simulink model "testEmplanner_cs_old"  (R2021b)
settings: Solver=ode5  StartTime=0.0  StopTime=60  FixedStep=1/1000  RelTol=1e-3
PreLoadFcn:
  | mbxruntime.callbacks.PreLoadFcn(bdroot);
PostLoadFcn:
  | mbxruntime.callbacks.PostLoadFcn(bdroot);
InitFcn:
  | mbxruntime.callbacks.InitFcn(bdroot);
StartFcn:
  | mbxruntime.callbacks.StartFcn(bdroot);
StopFcn:
  | mbxruntime.callbacks.StopFcn(bdroot);
model workspace (MAT data in the model file):
  mbox_table : object (value not decoded)
  model_closed = 0
  sim_status = 0
values from neighbouring files (symbols this model uses):
  c_factor = 43.75    [emplanner_init.m]
  cf = -175016    [emplanner_init.m]
  cr = -130634    [emplanner_init.m]
  global_path_x = [-1.1448 -0.145417744933 0.852705365581 1.84955224935 2.84511712279 3.83939835808 4.83239585569 5.82411007764 6.81454169183 7.80369144113 8.79156009523 9.77814843293 ... (3001 elements, 3001x1)]    [global_path.mat]
  global_path_y = [14.6488 14.6488 14.6488 14.6488 14.6488 14.6488 14.6488 14.6488 14.6488 14.6488 14.6488 14.6488 ... (3001 elements, 3001x1)]    [global_path.mat]
  KD_PID_distance = 0.0    (= 0)    [emplanner_init.m]
  KD_PID_speed = 0    [emplanner_init.m]
  KI_PID_distance = 0.0    (= 0)    [emplanner_init.m]
  KI_PID_speed = 0    [emplanner_init.m]
  KP_PID_distance = 0.5    [emplanner_init.m]
  KP_PID_speed = 1.8    [emplanner_init.m]
  la = 1.265    [emplanner_init.m]
  lb = 2.947-1.265    (= 1.682)    [emplanner_init.m]
  LQR_K1 = k(:,1)'    [emplanner_init.m]
  LQR_K2 = k(:,2)'    [emplanner_init.m]
  LQR_K3 = k(:,3)'    [emplanner_init.m]
  LQR_K4 = k(:,4)'    [emplanner_init.m]
  m = 2020    [emplanner_init.m]
  rack_displacement = [-39.14 , -37.2 , -35.29 , -33.43 , -31.6 , -29.81 , -28.06 , -26.34 , -24.66 ,      -23.01 , -21.38 , -19.79 , -18.23 , -16.69 , -15.18 , -13.7 , -12.23 , -10.8 , -9.38 , -7.98 ,     -6.61 , -5.25 , -3.91 , -2.59 , -1.29 , 0 , 1.27 , 2.54 , 3.78 , 5.02 , 6.24 , 7.46 , 8.66 ,      9.86 , 11.05 , 12.24 , 13.41 , 14.59 , 15.76 , 16.92 , 18.09 , 19.25 , 20.42 , 21.59 , 22.76 ,      23.93 , 25.11 , 26 ...(+26 chars)    [emplanner_init.m]
  right_wheel_ground = [-70 ,-67.2 , -64.4 , -61.6 , -58.8 , -56 , -53.2 , -50.4 , -47.6 , -44.8 , -42 ,      -39.2 , -36.4 , -33.6 , -30.8 , -28 , -25.2 , -22.4 , -19.6 , -16.8 , -14 , -11.2 , -8.4 , -5.6 ,      -2.8 , 0 , 2.8 , 5.6 , 8.4 , 11.2 , 14 , 16.8 , 19.6 , 22.4 , 25.2 , 28 , 30.8 , 33.6 , 36.4 ,      39.2 , 42 , 44.8 , 47.6 , 50.4 , 53.2 , 56 , 58.8 , 61.6 , 64.4 , 67.2 , 70 ]    [emplanner_init.m]
  vx_break_point = zeros(1,5000)    [emplanner_init.m]
undefined symbols (not defined in the file or in its folder): aubr, DiscIntNeverNeededParam, tablebr, vubr, warningInitialVelocity, x0
libraries: simulink x19, PreScanSimulinkLibrary x17, simulink_extras x6, Solver_SF x1
(part 11 of 14)

== matlab function testEmplanner_cs_old/Audi_A8_Sedan_1/decision&planning module/EM Planner/obs/MATLAB Function ==
  data: obs_x_set_gcs input; static_obs_x_set output; obs_y_set_gcs input; obs_heading_set_gcs input; obs_velocity_set_gcs input; static_obs_y_set output; dynamic_obs_x_set output; dynamic_obs_y_set output; dynamic_obs_vx_set output; dynamic_obs_vy_set output
function [static_obs_x_set,static_obs_y_set,dynamic_obs_x_set,dynamic_obs_y_set,dynamic_obs_vx_set,dynamic_obs_vy_set]...
	= fcn(obs_x_set_gcs,obs_y_set_gcs,obs_heading_set_gcs,obs_velocity_set_gcs)
%该函数将分类静态障碍物和动态障碍物
%输出初始化
n = 32;
static_obs_x_set = ones(n,1) * nan; 
static_obs_y_set = ones(n,1) * nan; 
dynamic_obs_x_set = ones(n,1) * nan; 
dynamic_obs_y_set = ones(n,1) * nan; 
dynamic_obs_vx_set = ones(n,1) * nan; 
dynamic_obs_vy_set = ones(n,1) * nan; 

count_static = 1;
count_dynamic = 1;

for i = 1 : length(obs_x_set_gcs)
	if isnan(obs_velocity_set_gcs(i))
		break;
	end
	if abs(obs_velocity_set_gcs(i)) < 0.1 
		static_obs_x_set(count_static) = obs_x_set_gcs(i); 
		static_obs_y_set(count_static) = obs_y_set_gcs(i);
		count_static = count_static + 1;
	else
		dynamic_obs_x_set(count_dynamic) = obs_x_set_gcs(i); 
		dynamic_obs_y_set(count_dynamic) = obs_y_set_gcs(i);
		dynamic_obs_vx_set(count_dynamic) = obs_velocity_set_gcs(i)*cos(obs_heading_set_gcs(i));
		dynamic_obs_vy_set(count_dynamic) = obs_velocity_set_gcs(i)*sin(obs_heading_set_gcs(i));
		count_dynamic = count_dynamic + 1;
	end
end

== matlab function testEmplanner_cs_old/Audi_A8_Sedan_1/decision&planning module/EM Planner/obs/MATLAB Function5 ==
  data: x_set input; match_point_index_set output; y_set input; frenet_path_x input; frenet_path_y input; frenet_path_heading input; frenet_path_kappa input; proj_x_set output; proj_y_set output; proj_heading_set output; proj_kappa_set output
function [match_point_index_set,proj_x_set,proj_y_set,proj_heading_set,proj_kappa_set] = ...
	fcn(x_set,y_set,frenet_path_x,frenet_path_y,frenet_path_heading,frenet_path_kappa)
	
%该函数将批量计算x_set,y_set中(x,y) 在frenet坐标系下的投影信息
%输入： x_set，y_set 待投影的点的集合
	%x_set,y_set,frenet_path_x,frenet_path_y,frenet_path_heading,frenet_path_kappa
	%曲线在直角坐标系下的x,y,heading,kappa
%输出：math_point_index_set 匹配点在frenet_path下的编号的集合（即从全局路径的第一个点开始数，第几个点是匹配点）

%由于事先不知道x_set中有多少个点需要投影，因此事先声明一个最大数量的点作为缓冲

n = 128;
%并且不知道投影点的数量，所以也不知道输出的数量，因此输出也要做缓冲，用nan表示不存在的点
%初始化输出最多为128个点。
%输出初始化
match_point_index_set = ones(n,1) * nan;
proj_x_set = ones(n,1) * nan;
proj_y_set = ones(n,1) * nan;
proj_heading_set = ones(n,1) * nan;
proj_kappa_set = ones(n,1) * nan;

%找匹配点，需要利用上一个周期的结果作为下一个周期遍历的起点，因此需要声明两个全局变量
persistent is_first_run;
persistent pre_match_point_index_set;
persistent pre_frenet_path_x;
persistent pre_frenet_path_y;
persistent pre_frenet_path_heading;
persistent pre_frenet_path_kappa;

%算法主函数入口

if isempty(is_first_run)
	% 该if分支表示函数首次运行
	is_first_run = 0; %赋值
	pre_frenet_path_x = frenet_path_x;
	pre_frenet_path_y = frenet_path_y;
	pre_frenet_path_heading = frenet_path_heading;
	pre_frenet_path_kappa = frenet_path_kappa;
	%记录首次运行计算的匹配点的结果供下个周期运行，先初始化
	pre_match_point_index_set = ones(n,1) * nan;
	
	%对x_set,y_set的点做遍历，找到他们的匹配点
	for i = 1 : length(x_set)
        if isnan(x_set(i))
            break;
        end
		%首次运行时，没有任何提示，只能从frenet_path的第一个点开始找
		start_search_index = 1;
		%声明increa_count,用于表示在遍历时distance连续增大的次数
		increase_count = 0;
		%开始遍历
		min_distance = inf;
		for j = start_search_index : length(frenet_path_x)
			distance = (x_set(i) - frenet_path_x(j))^2 + (y_set(i) - frenet_path_y(j))^2;
			%处理最小值
			if distance < min_distance
				min_distance = distance;
				match_point_index_set(i) = j; %math_point_index_set存放匹配点的序号
				increase_count = 0;
			else
				increase_count = increase_count + 1;
			end
			% 如果连续distanc增加50次,就不要再遍历了，节省时间
			if increase_count > 50 
				break;
			end	
		end
		%如何通过匹配点计算投影点，参考《自动驾驾驶控制算法第七讲》
		%或者《自动驾驶决策规划算法》第一章第三节
		
		%取出匹配点的编号
		match_point_index = match_point_index_set(i);
		
		%取出匹配点信息
		match_point_x = frenet_path_x(match_point_index);
		match_point_y = frenet_path_y(match_point_index);
		match_point_heading = frenet_path_heading(match_point_index);
		match_point_kappa = frenet_path_kappa(match_point_index);
		
		% 计算匹配点的位置向量和方向向量
		vector_match_point = [match_point_x;match_point_y];%位置向量
		vector_match_point_direction = [cos(match_point_heading);sin(match_point_heading)];%方向向量，全局坐标系下（大地坐标系）
		
		%声明待投影点的位矢
		vector_r = [x_set(i);y_set(i)];
		
		%通过匹配点计算投影点
		vector_d = vector_r - vector_match_point;
		ds = vector_d' * vector_match_point_direction;
		vector_proj_point = vector_match_point + vector_match_point_direction *ds;
		proj_heading = match_point_heading + match_point_kappa * ds;
		proj_kappa = match_point_kappa;
		
		%计算结果输出 
		proj_x_set(i) = vector_proj_point(1);
		proj_y_set(i) = vector_proj_point(2);
		proj_heading_set(i) = proj_heading;
		proj_kappa_set(i) = proj_kappa;
	end
	
	%匹配点的计算结果保存，供下一个周期使用
	pre_match_point_index_set = match_point_index_set;
else
	% 此分支不是首次运行
	
	%对每个x_set上的点做处理
	for i = 1 : length(x_set)
		%不是首次运行，对于点x_set(i),y_set(i)来说，start_search_index = pre_match_point_index_set(i)
		start_search_index = pre_match_point_index_set(i);%上个周期匹配点的编号作为本周期搜索的起点
		
        %
        % 对于障碍物的检测而言，当感知第一次检测到障碍物时，算法并不是首次运行，此时
        % pre_match_point_set的值是nan，如果还用上一个时刻的结果作为本周期搜索的起点
        % 必然会出问题，所以要修改
        % 声明 increase_count_limit
        increase_count_limit = 5;
        if isnan(start_search_index)
	        % 没有上个周期的结果，那么就不能只检查5次
	        increase_count_limit = 50;
	        % 搜索的起点也要设为 1
	        start_search_index = 1;
        end
		%声明increa_count,用于表示在遍历时distance连续增大的次数
		increase_count = 0;
		%开始遍历
		
		%这里多了一个步骤，判断遍历的方向
		%计算上个周期匹配点的位失
		vector_pre_match_point = [pre_frenet_path_x(start_search_index); pre_frenet_path_y(start_search_index)];
		vector_pre_match_point_direction = ...
			[cos(pre_frenet_path_heading(start_search_index));sin(pre_frenet_path_heading(start_search_index))];
		
		% 判断遍历的方向
		flag = ([x_set(i);y_set(i)] - vector_pre_match_point)' * vector_pre_match_point_direction;
		
		min_distance = inf;
		
		if flag > 0.001 
			for j = start_search_index : length(frenet_path_x)
				distance = (x_set(i) - frenet_path_x(j))^2 + (y_set(i) - frenet_path_y(j))^2;
				%处理最小值
				if distance < min_distance
					min_distance = distance;
					match_point_index_set(i) = j; %math_point_index_set存放匹配点的序号
					increase_count = 0;
				else
					increase_count = increase_count + 1;
				end
				% 如果连续distanc增加increase_count_limit次,就不要再遍历了，节省时间
				if increase_count > increase_count_limit
					break;
				end
			end
		elseif flag < -0.001
			for j = start_search_index :-1: 1
				distance = (x_set(i) - frenet_path_x(j))^2 + (y_set(i) - frenet_path_y(j))^2;
				%处理最小值
				if distance < min_distance
					min_distance = distance;
					match_point_index_set(i) = j; %math_point_index_set存放匹配点的序号
					increase_count = 0;
				else
					increase_count = increase_count + 1;
				end
				% 如果连续distanc增加50次,就不要再遍历了，节省时间
				if increase_count > increase_count_limit 
					break;
				end
			end
		else
			match_point_index_set(i) = start_search_index;
		end
			
		%如何通过匹配点计算投影点，参考《自动驾驾驶控制算法第七讲》
		%或者《自动驾驶决策规划算法》第一章第三节
		
		%取出匹配点的编号
		match_point_index = match_point_index_set(i);
		
		%取出匹配点信息
		match_point_x = frenet_path_x(match_point_index);
		match_point_y = frenet_path_y(match_point_index);
		match_point_heading = frenet_path_heading(match_point_index);
		match_point_kappa = frenet_path_kappa(match_point_index);
		
		% 计算匹配点的位置向量和方向向量
		vector_match_point = [match_point_x;match_point_y];%位置向量
		vector_match_point_direction = [cos(match_point_heading);sin(match_point_heading)];%方向向量
		
		%声明待投影点的位矢
		vector_r = [x_set(i);y_set(i)];
		
		%通过匹配点计算投影点
		vector_d = vector_r - vector_match_point;
		ds = vector_d' * vector_match_point_direction;
		vector_proj_point = vector_match_point + ds * vector_match_point_direction;
		proj_heading = match_point_heading + match_point_kappa * ds;
		proj_kappa = match_point_kappa;
		
		%计算结果输出 
		proj_x_set(i) = vector_proj_point(1);
		proj_y_set(i) = vector_proj_point(2);
		proj_heading_set(i) = proj_heading;
		proj_kappa_set(i) = proj_kappa;
	end
	
	%匹配点的计算结果保存，供下一个周期使用
	pre_match_point_index_set = match_point_index_set;
	pre_frenet_path_x = frenet_path_x;
	pre_frenet_path_y = frenet_path_y;
	pre_frenet_path_heading = frenet_path_heading;
	pre_frenet_path_kappa = frenet_path_kappa;
end

== matlab function testEmplanner_cs_old/Audi_A8_Sedan_1/decision&planning module/EM Planner/obs/obs filter ==
  data: host_x input; obs_x_set_final output; host_y input; host_heading_xy input; obs_x_set_gcs input; obs_y_set_gcs input; obs_heading_set_gcs input; obs_velocity_set_gcs input; obs_y_set_final output; obs_velocity_set_final output; obs_heading_set_final output
function [obs_x_set_final,obs_y_set_final,obs_velocity_set_final,obs_heading_set_final] = fcn(host_x,host_y,host_heading_xy, ...
	obs_x_set_gcs,obs_y_set_gcs,obs_heading_set_gcs,obs_velocity_set_gcs)
% 该函数将筛选障碍物，纵向[-10,60] 横向[-25,25]的障碍物才会被考虑
% 该函数只是一种单车道的临时办法，考虑到多车道情况，即使障碍物距离较远也应该考虑
% EM Planner 完全体是多车道并行计算的，每个车道都生成参考线后并行计算出多条轨迹，然后再选择最优轨迹作为输出
% 传感器最多可以识别32个障碍物
n = 32;
% 输出初始化

obs_x_set_final = ones(n,1)*nan;
obs_y_set_final = ones(n,1)*nan;
obs_velocity_set_final = ones(n,1)*nan;
obs_heading_set_final = ones(n,1)*nan;
count = 1;
for i = 1 : length(obs_x_set_gcs)
	if isnan(obs_x_set_gcs(i))
		break;
	end
	%自车的heading的方向向量与法向量
	tor = [cos(host_heading_xy);sin(host_heading_xy)];
	nor = [-sin(host_heading_xy);cos(host_heading_xy)];
	% 障碍物与自车的距离向量
	vetor_obs = [obs_x_set_gcs(i);obs_y_set_gcs(i)] - [host_x;host_y];
	% 障碍物距离自车的纵向距离
	lon_distance = vetor_obs' * tor;
	% 障碍物距离自车的横向距离
	lat_distance = vetor_obs' * nor;
	
	if (lon_distance < 60) && (lon_distance > -10) && (lat_distance > -25) && (lat_distance < 25)
		obs_x_set_final(count) = obs_x_set_gcs(i);
		obs_y_set_final(count) = obs_y_set_gcs(i);
		obs_heading_set_final(count) = obs_heading_set_gcs(i);
		obs_velocity_set_final(count) = obs_velocity_set_gcs(i);
		count = count + 1;
	end
end

== matlab function testEmplanner_cs_old/Audi_A8_Sedan_1/decision&planning module/EM Planner/path and speed merge ==
  data: s input; trajectory_x output; s_dot input; s_dot2 input; relative_time input; current_time input; path_s input; trajectory_x_init input; trajectory_y_init input; trajectory_heading_init input; trajectory_kappa_init input; trajectory_y output; trajectory_heading output; trajectory_kappa output; trajectory_speed output; trajectory_accel output; trajectory_time output
function [trajectory_x,trajectory_y,trajectory_heading,trajectory_kappa,trajectory_speed,trajectory_accel,trajectory_time] = ...
    fcn(s,s_dot,s_dot2,relative_time,current_time,path_s,trajectory_x_init,trajectory_y_init,trajectory_heading_init,trajectory_kappa_init)
% 该函数将合并path和speed
% 由于path 是 60个点，speed 有 401个点，合并后，path和speed有401个点，因此需要做插值
n = 401;
trajectory_x = zeros(n,1);
trajectory_y = zeros(n,1);
trajectory_heading = zeros(n,1);
trajectory_kappa = zeros(n,1);
trajectory_speed = zeros(n,1);

trajectory_accel = zeros(n,1);
index = 1;
% 由于trajectory_x_init中不是所有的值都有效，(有nan) 所以要找到有效值的范围
while ~isnan(trajectory_x_init(index)) 
    index = index + 1;
end
index = index - 1;
trajectory_time = zeros(n,1);
for i = 1:n-1
    %interp1 线性插值
    % 若 x = [1,2] y = [3,4]
    %interp1(x,y,1.5) 会得到3.5
    %interp1 的缺点是 在端点或超过端点的，结果为nan
    % interp1(x,y,2) 不会等于4 而是会等于nan
    % interp1(x,y,6) 也会等于nan，所以在端点处要单独处理
    trajectory_x(i) = interp1(path_s(1:index),trajectory_x_init(1:index),s(i));
    trajectory_y(i) = interp1(path_s(1:index),trajectory_y_init(1:index),s(i));
    trajectory_heading(i) = interp1(path_s(1:index),trajectory_heading_init(1:index),s(i));
    trajectory_kappa(i) = interp1(path_s(1:index),trajectory_kappa_init(1:index),s(i));
    trajectory_time(i) = relative_time(i) + current_time;%速度规划会得到相对时间，转换成绝对时间
    trajectory_speed(i) = s_dot(i);
    trajectory_accel(i) = s_dot2(i);
end
% 端点单独处理
trajectory_x(end) = trajectory_x_init(end);
trajectory_y(end) = trajectory_y_init(end);
trajectory_heading(end) = trajectory_heading_init(end);
trajectory_kappa(end) = trajectory_kappa_init(end);
trajectory_time(end) = relative_time(end) + current_time;
trajectory_speed(end) = s_dot(end);
trajectory_accel(end) = s_dot2(end);

== matlab function testEmplanner_cs_old/Audi_A8_Sedan_2/PathFollower_Preview_1/LateralController/Calculate delta steering error/eml_delta_steering_error ==
  data: v_x_vehicle input; v_x_vehicle_Min input; t_Preview_LatCtrl input; delta_steeringwheeltotal output; v_y_vehicle input; yawrate_vehicle input; CorneringStiffness_Tyres_Front input; CorneringStiffness_Tyres_Rear input; m_vehicle_total input; inertia_z_vehicle_total input; e_Lat input size=10; Pos_x_CoG_Vehicle input; wheelbase input; RefreshCounter parameter
function delta_steeringwheeltotal = eml_delta_steering_error(v_x_vehicle,v_x_vehicle_Min,t_Preview_LatCtrl,v_y_vehicle,yawrate_vehicle,CorneringStiffness_Tyres_Front,CorneringStiffness_Tyres_Rear,m_vehicle_total,inertia_z_vehicle_total,e_Lat,Pos_x_CoG_Vehicle,wheelbase,RefreshCounter)

delta_steeringwheeltotal = emlfcn_delta_steering_error(v_x_vehicle,v_x_vehicle_Min,t_Preview_LatCtrl,v_y_vehicle,yawrate_vehicle,CorneringStiffness_Tyres_Front,CorneringStiffness_Tyres_Rear,m_vehicle_total,inertia_z_vehicle_total,e_Lat,Pos_x_CoG_Vehicle,wheelbase,RefreshCounter);

% end function

== matlab function testEmplanner_cs_old/Audi_A8_Sedan_1/decision&planning module/EM Planner/plot ==
  data: dp_s input; dp_l input; qp_s input; qp_l input; l_min input; l_max input; obs_s_set input; obs_l_set input; start_s input; start_l input; start_dl input
function  fcn(dp_s,dp_l,qp_s,qp_l,l_min,l_max,obs_s_set,obs_l_set,start_s,start_l,start_dl)
coder.extrinsic("plot","axis","figure","drawnow","cla","fill");

obs_length = 5;
obs_width = 2;
host_l = 6;
host_w = 1.63;
cla;
host_p1_l = start_l + sin(atan(start_dl)) * host_l /2 + host_w/2 * cos(atan(start_dl));
host_p1_s = start_s + cos(atan(start_dl)) * host_l /2 - host_w/2 * sin(atan(start_dl));
host_p2_l = start_l + sin(atan(start_dl)) * host_l /2 - host_w/2 * cos(atan(start_dl));
host_p2_s = start_s + cos(atan(start_dl)) * host_l /2 + host_w/2 * sin(atan(start_dl));
host_p3_l = start_l - sin(atan(start_dl)) * host_l /2 + host_w/2 * cos(atan(start_dl));
host_p3_s = start_s - cos(atan(start_dl)) * host_l /2 - host_w/2 * sin(atan(start_dl));
host_p4_l = start_l - sin(atan(start_dl)) * host_l /2 - host_w/2 * cos(atan(start_dl));
host_p4_s = start_s - cos(atan(start_dl)) * host_l /2 + host_w/2 * sin(atan(start_dl));
host_area_x = [host_p1_s;host_p2_s;host_p4_s;host_p3_s];
host_area_y = [host_p1_l;host_p2_l;host_p4_l;host_p3_l];
fill(host_area_x,host_area_y,[0 1 1]);
hold on
plot(dp_s,dp_l,'r');

plot(qp_s,qp_l,'b');
plot(dp_s,l_min,dp_s,l_max);
axis([-8 70 -10 10]);

for i = 1:length(obs_s_set)
    if isnan(obs_s_set(i))
        break;
    end
    obs_p1_s = obs_s_set(i) + obs_length/2;
    obs_p1_l = obs_l_set(i) + obs_width/2;
    obs_p2_s = obs_s_set(i) + obs_length/2;
    obs_p2_l = obs_l_set(i) - obs_width/2;
    obs_p3_s = obs_s_set(i) - obs_length/2;
    obs_p3_l = obs_l_set(i) + obs_width/2;
    obs_p4_s = obs_s_set(i) - obs_length/2;
    obs_p4_l = obs_l_set(i) - obs_width/2;
    obs_area_s = [obs_p1_s;obs_p2_s;obs_p4_s;obs_p3_s];
    obs_area_l = [obs_p1_l;obs_p2_l;obs_p4_l;obs_p3_l];
    fill(obs_area_s,obs_area_l,[0 0 0]);
end

== matlab function testEmplanner_cs_old/Audi_A8_Sedan_1/decision&planning module/EM Planner/simple speed qp planning ==
  data: plan_start_s_dot input; s_init output; plan_start_s_dot2 input; s_end input; recommend_T input; s_dot_init output; s_dot2_init output; relative_time_init output
function [s_init,s_dot_init,s_dot2_init,relative_time_init] = fcn(plan_start_s_dot,plan_start_s_dot2,s_end,recommend_T)
%简单速度二次规划
coder.extrinsic("quadprog")
n = 51;
s_init = zeros(n,1);
s_dot_init = zeros(n,1);
s_dot2_init = zeros(n,1);
relative_time_init = zeros(n,1);

Aeq = zeros(3*n,2*n - 2);
beq = zeros(2*n - 2,1);
lb = ones(3*n,1);
ub = lb;
dt = recommend_T/(n-1);
A_sub =[1,0;
        dt,1;
        (1/3)*dt^2,(1/2)*dt;
        -1,0;
        0,-1;
        (1/6)*dt^2,dt/2];
for i = 1:n - 1
    Aeq(3*i-2:3*i+3,2*i-1:2*i) = A_sub;
end

for i = 1:n
   lb(3*i - 2) = -inf;
   lb(3*i - 1) = 0;
   lb(3*i) = -8;
   ub(3*i - 2) = inf;
   ub(3*i - 1) = 50;
   ub(3*i) = 2;
end
lb(1) = 0;
lb(2) = plan_start_s_dot;
lb(3) = plan_start_s_dot2;
ub(1) = lb(1);
ub(2) = lb(2);
ub(3) = lb(3);
lb(3*n - 2) = s_end;
ub(3*n - 2) = s_end;
A3 = zeros(3*n,3*n);
A4 = zeros(3*n,n - 1);
A4_sub =[0;0;1;0;0;-1];
for i = 1:n - 1
   A3(3*i,3*i) = 1;
   A4(3*i-2:3*i+3,i:i) = A4_sub;
end
A3(3*n,3*n) = 1;
H = A3 + 100*(A4*A4');
H = 2*H;
f = zeros(3*n,1);
X = quadprog(H,f,[],[],Aeq',beq,lb,ub);
for i = 1:n
   s_init(i) = X(3*i - 2);
   s_dot_init(i) = X(3*i - 1);
   s_dot2_init(i) = X(3*i);
   relative_time_init(i) = (i - 1)*dt;
end

== matlab function testEmplanner_cs_old/Audi_A8_Sedan_1/decision&planning module/EM Planner/stitch trajectory ==
  data: trajectory_x input; trajectory_x_final output; trajectory_y input; trajectory_heading input; trajectory_kappa input; trajectory_speed input; trajectory_accel input; trajectory_time input; stitch_x input; stitch_y input; stitch_heading input; stitch_kappa input; stitch_speed input; stitch_accel input; stitch_time input; trajectory_y_final output; trajectory_heading_final output; trajectory_kappa_final output; trajectory_speed_final output; trajectory_accel_final output; trajectory_time_final output
function [trajectory_x_final,trajectory_y_final,trajectory_heading_final,trajectory_kappa_final,...
          trajectory_speed_final,trajectory_accel_final,trajectory_time_final] = fcn(trajectory_x,...
          trajectory_y,trajectory_heading,trajectory_kappa,trajectory_speed,trajectory_accel,trajectory_time,...
          stitch_x,stitch_y,stitch_heading,stitch_kappa,stitch_speed,stitch_accel,stitch_time)
% 轨迹拼接，把stitch trajectory 拼到规划完成的轨迹上
n = 401 + 20;
trajectory_x_final = zeros(n,1);
trajectory_y_final = zeros(n,1);
trajectory_heading_final = zeros(n,1);
trajectory_kappa_final = zeros(n,1);
trajectory_speed_final = zeros(n,1);
trajectory_accel_final = zeros(n,1);
trajectory_time_final = zeros(n,1);

trajectory_x_final = [stitch_x;trajectory_x];
trajectory_y_final = [stitch_y;trajectory_y];
trajectory_heading_final = [stitch_heading;trajectory_heading];
trajectory_kappa_final = [stitch_kappa;trajectory_kappa];
trajectory_speed_final = [stitch_speed;trajectory_speed];
trajectory_accel_final = [stitch_accel;trajectory_accel];
trajectory_time_final = [stitch_time;trajectory_time];

== matlab function testEmplanner_cs_old/Audi_A8_Sedan_1/decision&planning module/EM Planner2/simple speed qp planning ==
  data: plan_start_s_dot input; s_init output; plan_start_s_dot2 input; s_end input; recommend_T input; s_dot_init output; s_dot2_init output; relative_time_init output
function [s_init,s_dot_init,s_dot2_init,relative_time_init] = fcn(plan_start_s_dot,plan_start_s_dot2,s_end,recommend_T)
%简单速度二次规划
coder.extrinsic("quadprog")
n = 51;
s_init = zeros(n,1);
s_dot_init = zeros(n,1);
s_dot2_init = zeros(n,1);
relative_time_init = zeros(n,1);

Aeq = zeros(3*n,2*n - 2);
beq = zeros(2*n - 2,1);
lb = ones(3*n,1);
ub = lb;
dt = recommend_T/(n-1);
A_sub =[1,0;
        dt,1;
        (1/3)*dt^2,(1/2)*dt;
        -1,0;
        0,-1;
        (1/6)*dt^2,dt/2];
for i = 1:n - 1
    Aeq(3*i-2:3*i+3,2*i-1:2*i) = A_sub;
end

for i = 1:n
   lb(3*i - 2) = -inf;
   lb(3*i - 1) = 0;
   lb(3*i) = -8;
   ub(3*i - 2) = inf;
   ub(3*i - 1) = 50;
   ub(3*i) = 2;
end
lb(1) = 0;
lb(2) = plan_start_s_dot;
lb(3) = plan_start_s_dot2;
ub(1) = lb(1);
ub(2) = lb(2);
ub(3) = lb(3);
lb(3*n - 2) = s_end;
ub(3*n - 2) = s_end;
A3 = zeros(3*n,3*n);
A4 = zeros(3*n,n - 1);
A4_sub =[0;0;1;0;0;-1];
for i = 1:n - 1
   A3(3*i,3*i) = 1;
   A4(3*i-2:3*i+3,i:i) = A4_sub;
end
A3(3*n,3*n) = 1;
H = A3 + 100*(A4*A4');
H = 2*H;
f = zeros(3*n,1);
X = quadprog(H,f,[],[],Aeq',beq,lb,ub);
for i = 1:n
   s_init(i) = X(3*i - 2);
   s_dot_init(i) = X(3*i - 1);
   s_dot2_init(i) = X(3*i);
   relative_time_init(i) = (i - 1)*dt;
end

== matlab function testEmplanner_cs_old/Audi_A8_Sedan_1/decision&planning module/EM Planner2/stitch trajectory ==
  data: trajectory_x input; trajectory_x_final output; trajectory_y input; trajectory_heading input; trajectory_kappa input; trajectory_speed input; trajectory_accel input; trajectory_time input; stitch_x input; stitch_y input; stitch_heading input; stitch_kappa input; stitch_speed input; stitch_accel input; stitch_time input; trajectory_y_final output; trajectory_heading_final output; trajectory_kappa_final output; trajectory_speed_final output; trajectory_accel_final output; trajectory_time_final output
function [trajectory_x_final,trajectory_y_final,trajectory_heading_final,trajectory_kappa_final,...
          trajectory_speed_final,trajectory_accel_final,trajectory_time_final] = fcn(trajectory_x,...
          trajectory_y,trajectory_heading,trajectory_kappa,trajectory_speed,trajectory_accel,trajectory_time,...
          stitch_x,stitch_y,stitch_heading,stitch_kappa,stitch_speed,stitch_accel,stitch_time)
% 轨迹拼接，把stitch trajectory 拼到规划完成的轨迹上
n = 401 + 20;
trajectory_x_final = zeros(n,1);
trajectory_y_final = zeros(n,1);
trajectory_heading_final = zeros(n,1);
trajectory_kappa_final = zeros(n,1);
trajectory_speed_final = zeros(n,1);
trajectory_accel_final = zeros(n,1);
trajectory_time_final = zeros(n,1);

trajectory_x_final = [stitch_x;trajectory_x];
trajectory_y_final = [stitch_y;trajectory_y];
trajectory_heading_final = [stitch_heading;trajectory_heading];
trajectory_kappa_final = [stitch_kappa;trajectory_kappa];
trajectory_speed_final = [stitch_speed;trajectory_speed];
trajectory_accel_final = [stitch_accel;trajectory_accel];
trajectory_time_final = [stitch_time;trajectory_time];

== matlab function testEmplanner_cs_old/Audi_A8_Sedan_1/decision&planning module/referenceline provider/MATLAB Function3 ==
  data: path_x input; path_heading output; path_y input; path_kappa output
function [path_heading,path_kappa] = fcn(path_x,path_y)
%该函数将计算path的切线方向与x轴的夹角和曲率
%输入：path_x,path_y路径的坐标（全局坐标系下）
%输出：path_heading,path_kappa 路径的heading和曲率
%原理：heading = arctan(dy/dx)
%  kappa = dheading /ds
%  ds = (dx^2 + dy^2)^0.5


%注意，角度的多值性会带来很大的麻烦，需要慎重处理
%例如： x与 x+2*pi代表同一个角度，这种多值性在曲率计算的时候会带来麻烦
%比如： 原本是（0.1 -（-0.1））/ ds,但是如果计算出得-0.1多了一个2*pi
%kappa 就等于(0.1 -(-0.1 + 2*pi)) /ds 曲率就会变得非常大
%还有若采用中点欧拉法计算heading时，即使用 (y2 - y1) / (x2 - x1)的反正切计算一个角度，用(y1 - y0)/(x1 - x0)的反正切
%又计算了一个角度，然后加起来除以2，如果精确值是(a1 + a2)/2,但是最终计算结果可能是(a1 + a2 + 2pi) / 2
%还有tan(x) = tan(x + pi） 所以 arctan(tan(x)) 可能等于x,也可能等于x + pi
%角度的处理非常麻烦，而且角度处理不当往往是许多奇怪错误的源头
%

dx = diff(path_x);
dy = diff(path_y);%计算差分

%用中点欧拉法要比向前欧拉法和向后欧拉法要更精确，但是也可能计算出的结果比精确值多一个pi
%在这里对dx,dy做中点欧拉法，使用四象限反正切计算角度

dx_pre = [dx(1);dx];
dx_after = [dx;dx(end)];
dx_final = (dx_pre + dx_after) / 2;

dy_pre = [dy(1);dy];
dy_after = [dy;dy(end)];
dy_final = (dy_pre + dy_after) / 2;

ds_final = sqrt(dx_final.^2 + dy_final.^2);
path_heading = atan2(dy_final,dx_final);

%atan2(b，a)：4象限反正切，

%　　　　计算b/a对应的反正切值，求点(a，b)对应的角
% 　　　　　(a，b)位于第一象限时，atan2(b，a)取值  0 ~ pi/2
% 　　　　　(a，b)位于第二象限时，atan2(b，a)取值  pi/2 ~ pi
% 　　　　　(a，b)位于第三象限时，atan2(b，a)取值   -pi ~ -pi/2
% 　　　　　(a，b)位于第四象限时，atan2(b，a)取值   -pi/2 ~ 0
%

%中点欧拉法
dheading = diff(path_heading);%差分，size变成length(path_heading) - 1
dheading_pre = [dheading(1);dheading]; %插入一个首元素
dheading_after = [dheading;dheading(end)]; %插入一个尾元素
dheading_final = (dheading_pre + dheading_after) / 2;
%为了防止dheading出现一个2*pi的错误，假设真实的heading较小，用sin(dheading)近似dheading
path_kappa = sin(dheading_final)./ds_final;

== matlab function testEmplanner_cs_old/Audi_A8_Sedan_1/decision&planning module/referenceline provider/MATLAB Function4 ==
  data: referenceline_x_init input; referenceline_x output; referenceline_y_init input; w_cost_smooth input; w_cost_length input; w_cost_ref input; x_lb input; x_ub input; y_lb input; y_ub input; referenceline_y output
function [referenceline_x,referenceline_y] = ...
 	fcn(referenceline_x_init,referenceline_y_init,w_cost_smooth,w_cost_length,w_cost_ref,x_lb,x_ub,y_lb,y_ub)
 %该函数将平滑referenceline
 %使用二次规划算法
 %原理：
 %	0.5x'Hx + f'x = min 
 %约束条件:
 %	lb <= x <= ub
 %输入： referenceline_x_init,referenceline_y_init,未平滑的参考线
 %w_cost_smooth,w_cost_length,w_cost_ref 平滑代价，紧凑代价，几何相似代价权重系数
 %x_lb,x_ub,y_lb,y_ub 允许x,y变化的上下界
 %输出：referenceline_x,referenceline_y 平滑后的参考线
 
 %这里为了简化，不适用拼接算法
 %计算量问题通过调度器来解决，规划周期设置100ms，只要在100ms完成就可以了
 %如果到最后计算速度还是问题，再进行优化，目前暂时不适用拼接算法
 
 %simulink 无法直接使用自带的二次规划函数，需要从外部引入，执行下面命令
 
 coder.extrinsic("quadprog");
  %二次规划的形式
%   H1 = w_cost_smooth * (A1'*A1) + w_cost_length*(A2'*A2) + w_cost_ref * (A3'*A3)
%   f = -2 * w_cost_ref * referenceline_x 
%   x’H1x + f'x = 0.5 * x'(2H1)*x + f'x
%   A1 = [1 0 -2 0 1 0 
%            1 0 -2 0 1 
%              1  0 -2 0 1 
%                    .........
%  
%   A2 = [ 1 0 -1 0
%            1 0  -1 0 
%              1 0 -1 0
%                1 0  -1 0 
%                  ........
 
 %A3 为单位矩阵
 
 %设置求解矩阵的规模，因为参考线初始点一共181个，每个点有两个坐标，所以求解矩阵规模是362
 n = 181;
 %referenceline初始化
 referenceline_x = zeros(n,1);
 referenceline_y = zeros(n,1);
 
 
 A1 = zeros(2 * n - 4, 2 * n);
 A2 = zeros(2 * n - 2, 2 * n);
 A3 = eye(2 * n,2 * n);
 f = zeros(2 * n,1);
 lb = zeros(2 * n,1);
 ub = zeros(2 * n,1);
 persistent is_first_run;
 persistent pre_result_x;
 persistent pre_result_y;
 persistent pre_referenceline_x_init;
 persistent pre_referenceline_y_init;
 
 if isempty(is_first_run)
 	is_first_run = 0;
 	% 一个坐标具有两个值,f(2*i-1)是对应的x,f(2*i)是对应的y
 	for i = 1 : n
 		f(2*i - 1) = referenceline_x_init(i);
 		f(2*i) = referenceline_y_init(i);
 		lb(2*i-1) = f(2*i - 1) + x_lb;
 		ub(2*i-1) = f(2*i - 1) + x_ub;
 		lb(2*i) = f(2*i) + y_lb;
 		ub(2*i) = f(2*i) + y_ub;
 	end
 
 	for j = 1 : 2 : 2 * n - 5
 		A1(j,j) = 1;
 		A1(j,j+2) = -2;
 		A1(j,j+4) = 1;
 		A1(j+1,j+1) = 1;
 		A1(j+1,j+3) = -2;
 		A1(j+1,j+5) = 1;
 	end
 
 	for k = 1 : 2 :2 * n -3
 		A2(k,k) = 1;
 		A2(k,k+2) = -1;
 		A2(k+1,k+1) = 1;
 		A2(k+1,k+3) = -1;
 	end
 
 	H1 = w_cost_smooth * (A1'*A1)  + w_cost_length *(A2'*A2) + w_cost_ref * A3;
 	H = 2 * H1;
 	%用 referenceline的初值作为二次规划的迭代的起点,加速二次规划的过程
 	X0 = f;
 	f = -2 * w_cost_ref * f;
 	
 	%二次规划求解
 	X = quadprog(H,f,[],[],[],[],lb,ub,X0);
 	%将结果输出到referenceline中
 	for i = 1 : n 
 		referenceline_x(i) = X(2*i -1);
 		referenceline_y(i) = X(2*i);
 	end
 	pre_result_x = referenceline_x;
 	pre_result_y = referenceline_y;
 	pre_referenceline_x_init = referenceline_x_init;
 	pre_referenceline_y_init = referenceline_y_init;
 else
    if pre_referenceline_x_init(1) == referenceline_x_init(1) && ...
 		pre_referenceline_y_init(1) == referenceline_y_init(1) 
 		 %起点相同，可以认为本周期和上个周期reference_init 完全相同，直接使用
 		referenceline_x = pre_result_x;
 		referenceline_y = pre_result_y;
    else
        for i = 1 : n
 			f(2*i - 1) = referenceline_x_init(i);
 			f(2*i) = referenceline_y_init(i);
 			lb(2*i-1) = f(2*i - 1) + x_lb;
 			ub(2*i-1) = f(2*i - 1) + x_ub;
 			lb(2*i) = f(2*i) + y_lb;
 			ub(2*i) = f(2*i) + y_ub;
        end
 
 		for j = 1 : 2 : 2 * n - 5
 			A1(j,j) = 1;
 			A1(j,j+2) = -2;
 			A1(j,j+4) = 1;
 			A1(j+1,j+1) = 1;
 			A1(j+1,j+3) = -2;
 			A1(j+1,j+5) = 1;
 		end
 
        for k = 1 : 2 : 2*n -3
 			A2(k,k) = 1;
 			A2(k,k+2) = -1;
 			A2(k+1,k+1) = 1;
 			A2(k+1,k+3) = -1;
        end 	
 	    H1 = w_cost_smooth * (A1'*A1)  + w_cost_length *(A2'*A2) + w_cost_ref * A3;
 	    H = 2 * H1;
 	    %用 referenceline的初值作为二次规划的迭代的起点,加速二次规划的过程
 	    X0 = f ;
 	    f = -2 * w_cost_ref * f;
 	    
 	    %二次规划求解
 	    X = quadprog(H,f,[],[],[],[],lb,ub,X0);
 	    %将结果输出到referenceline中
 	    for i = 1 :n 
 		    referenceline_x(i) = X(2*i -1);
 		    referenceline_y(i) = X(2*i);
 	    end
 	    pre_result_x = referenceline_x;
 	    pre_result_y = referenceline_y;
 	    pre_referenceline_x_init = referenceline_x_init;
 	    pre_referenceline_y_init = referenceline_y_init;
    end
 end

== matlab function testEmplanner_cs_old/Audi_A8_Sedan_1/decision&planning module/Subsystem/MATLAB Function ==
  data: x_set input; match_point_index_set output; y_set input; frenet_path_x input; frenet_path_y input; frenet_path_heading input; frenet_path_kappa input; proj_x_set output; proj_y_set output; proj_heading_set output; proj_kappa_set output
function [match_point_index_set,proj_x_set,proj_y_set,proj_heading_set,proj_kappa_set] = ...
	fcn(x_set,y_set,frenet_path_x,frenet_path_y,frenet_path_heading,frenet_path_kappa)
	
%该函数将批量计算x_set,y_set中(x,y) 在frenet坐标系下的投影信息
%输入： x_set，y_set 待投影的点的集合
	%x_set,y_set,frenet_path_x,frenet_path_y,frenet_path_heading,frenet_path_kappa
	%曲线在直角坐标系下的x,y,heading,kappa
%输出：math_point_index_set 匹配点在frenet_path下的编号的集合（即从全局路径的第一个点开始数，第几个点是匹配点）

%由于事先不知道x_set中有多少个点需要投影，因此事先声明一个最大数量的点作为缓冲

n = 128;
%并且不知道投影点的数量，所以也不知道输出的数量，因此输出也要做缓冲，用nan表示不存在的点
%初始化输出最多为128个点。
%输出初始化
match_point_index_set = ones(n,1) * nan;
proj_x_set = ones(n,1) * nan;
proj_y_set = ones(n,1) * nan;
proj_heading_set = ones(n,1) * nan;
proj_kappa_set = ones(n,1) * nan;

%找匹配点，需要利用上一个周期的结果作为下一个周期遍历的起点，因此需要声明两个全局变量
persistent is_first_run;
persistent pre_match_point_index_set;
persistent pre_frenet_path_x;
persistent pre_frenet_path_y;
persistent pre_frenet_path_heading;
persistent pre_frenet_path_kappa;

%算法主函数入口

if isempty(is_first_run)
	% 该if分支表示函数首次运行
	is_first_run = 0; %赋值
	pre_frenet_path_x = frenet_path_x;
	pre_frenet_path_y = frenet_path_y;
	pre_frenet_path_heading = frenet_path_heading;
	pre_frenet_path_kappa = frenet_path_kappa;
	%记录首次运行计算的匹配点的结果供下个周期运行，先初始化
	pre_match_point_index_set = ones(n,1) * nan;
	
	%对x_set,y_set的点做遍历，找到他们的匹配点
	for i = 1 : length(x_set)
		%首次运行时，没有任何提示，只能从frenet_path的第一个点开始找
		start_search_index = 1;
		%声明increa_count,用于表示在遍历时distance连续增大的次数
		increase_count = 0;
		%开始遍历
		min_distance = inf;
		for j = start_search_index : length(frenet_path_x)
			distance = (x_set(i) - frenet_path_x(j))^2 + (y_set(i) - frenet_path_y(j))^2;
			%处理最小值
			if distance < min_distance
				min_distance = distance;
				match_point_index_set(i) = j; %math_point_index_set存放匹配点的序号
				increase_count = 0;
			else
				increase_count = increase_count + 1;
			end
			% 如果连续distanc增加50次,就不要再遍历了，节省时间
			if increase_count > 50 
				break;
			end	
		end
		%如何通过匹配点计算投影点，参考《自动驾驾驶控制算法第七讲》
		%或者《自动驾驶决策规划算法》第一章第三节
		
		%取出匹配点的编号
		match_point_index = match_point_index_set(i);
		
		%取出匹配点信息
		match_point_x = frenet_path_x(match_point_index);
		match_point_y = frenet_path_y(match_point_index);
		match_point_heading = frenet_path_heading(match_point_index);
		match_point_kappa = frenet_path_kappa(match_point_index);
		
		% 计算匹配点的位置向量和方向向量
		vector_match_point = [match_point_x;match_point_y];%位置向量
		vector_match_point_direction = [cos(match_point_heading);sin(match_point_heading)];%方向向量，全局坐标系下（大地坐标系）
		
		%声明待投影点的位矢
		vector_r = [x_set(i);y_set(i)];
		
		%通过匹配点计算投影点
		vector_d = vector_r - vector_match_point;
		ds = vector_d' * vector_match_point_direction;
		vector_proj_point = vector_match_point + ds * vector_match_point_direction;
		proj_heading = match_point_heading + match_point_kappa * ds;
		proj_kappa = match_point_kappa;
		
		%计算结果输出 
		proj_x_set(i) = vector_proj_point(1);
		proj_y_set(i) = vector_proj_point(2);
		proj_heading_set(i) = proj_heading;
		proj_kappa_set(i) = proj_kappa;
	end
	
	%匹配点的计算结果保存，供下一个周期使用
	pre_match_point_index_set = match_point_index_set;
else
	% 此分支不是首次运行
	
	%对每个x_set上的点做处理
	for i = 1 : length(x_set)
		%不是首次运行，对于点x_set(i),y_set(i)来说，start_search_index = pre_match_point_index_set(i)
		start_search_index = pre_match_point_index_set(i);%上个周期匹配点的编号作为本周期搜索的起点
		
		%声明increa_count,用于表示在遍历时distance连续增大的次数
		increase_count = 0;
		%开始遍历
		
		%这里多了一个步骤，判断遍历的方向
		%计算上个周期匹配点的位失
		vector_pre_match_point = [pre_frenet_path_x(start_search_index); pre_frenet_path_y(start_search_index)];
		vector_pre_match_point_direction = ...
			[cos(pre_frenet_path_heading(start_search_index));sin(pre_frenet_path_heading(start_search_index))];
		
		% 判断遍历的方向
		flag = ([x_set(i);y_set(i)] - vector_pre_match_point)' * vector_pre_match_point_direction;
		
		min_distance = inf;
		
		if flag > 0.001 
			for j = start_search_index : length(frenet_path_x)
				distance = (x_set(i) - frenet_path_x(j))^2 + (y_set(i) - frenet_path_y(j))^2;
				%处理最小值
				if distance < min_distance
					min_distance = distance;
					match_point_index_set(i) = j; %math_point_index_set存放匹配点的序号
					increase_count = 0;
				else
					increase_count = increase_count + 1;
				end
				% 如果连续distanc增加5次,就不要再遍历了，节省时间
				if increase_count > 5 
					break;
				end
			end
		elseif flag < -0.001
			for j = start_search_index :-1: 1
				distance = (x_set(i) - frenet_path_x(j))^2 + (y_set(i) - frenet_path_y(j))^2;
				%处理最小值
				if distance < min_distance
					min_distance = distance;
					match_point_index_set(i) = j; %math_point_index_set存放匹配点的序号
					increase_count = 0;
				else
					increase_count = increase_count + 1;
				end
				% 如果连续distanc增加50次,就不要再遍历了，节省时间
				if increase_count > 5 
					break;
				end
			end
		else
			match_point_index_set(i) = start_search_index;
		end
			
		%如何通过匹配点计算投影点，参考《自动驾驾驶控制算法第七讲》
		%或者《自动驾驶决策规划算法》第一章第三节
		
		%取出匹配点的编号
		match_point_index = match_point_index_set(i);
		
		%取出匹配点信息
		match_point_x = frenet_path_x(match_point_index);
		match_point_y = frenet_path_y(match_point_index);
		match_point_heading = frenet_path_heading(match_point_index);
		match_point_kappa = frenet_path_kappa(match_point_index);
		
		% 计算匹配点的位置向量和方向向量
		vector_match_point = [match_point_x;match_point_y];%位置向量
		vector_match_point_direction = [cos(match_point_heading);sin(match_point_heading)];%方向向量
		
		%声明待投影点的位矢
		vector_r = [x_set(i);y_set(i)];
		
		%通过匹配点计算投影点
		vector_d = vector_r - vector_match_point;
		ds = vector_d' * vector_match_point_direction;
		vector_proj_point = vector_match_point + ds * vector_match_point_direction;
		proj_heading = match_point_heading + match_point_kappa * ds;
		proj_kappa = match_point_kappa;
		
		%计算结果输出 
		proj_x_set(i) = vector_proj_point(1);
		proj_y_set(i) = vector_proj_point(2);
		proj_heading_set(i) = proj_heading;
		proj_kappa_set(i) = proj_kappa;
	end
	
	%匹配点的计算结果保存，供下一个周期使用
	pre_match_point_index_set = match_point_index_set;
	pre_frenet_path_x = frenet_path_x;
	pre_frenet_path_y = frenet_path_y;
	pre_frenet_path_heading = frenet_path_heading;
	pre_frenet_path_kappa = frenet_path_kappa;
end

== matlab function testEmplanner_cs_old/Audi_A8_Sedan_1/decision&planning module/Subsystem/MATLAB Function1 ==
  data: path_x input; path_heading output; path_y input; path_kappa output
function [path_heading,path_kappa] = fcn(path_x,path_y)
%该函数将计算path的切线方向与x轴的夹角和曲率
%输入：path_x,path_y路径的坐标（全局坐标系下）
%输出：path_heading,path_kappa 路径的heading和曲率
%原理：heading = arctan(dy/dx)
%  kappa = dheading /ds
%  ds = (dx^2 + dy^2)^0.5


%注意，角度的多值性会带来很大的麻烦，需要慎重处理
%例如： x与 x+2*pi代表同一个角度，这种多值性在曲率计算的时候会带来麻烦
%比如： 原本是（0.1 -（-0.1））/ ds,但是如果计算出得-0.1多了一个2*pi
%kappa 就等于(0.1 -(-0.1 + 2*pi)) /ds 曲率就会变得非常大
%还有若采用中点欧拉法计算heading时，即使用 (y2 - y1) / (x2 - x1)的反正切计算一个角度，用(y1 - y0)/(x1 - x0)的反正切
%又计算了一个角度，然后加起来除以2，如果精确值是(a1 + a2)/2,但是最终计算结果可能是(a1 + a2 + 2pi) / 2
%还有tan(x) = tan(x + pi） 所以 arctan(tan(x)) 可能等于x,也可能等于x + pi
%角度的处理非常麻烦，而且角度处理不当往往是许多奇怪错误的源头
%

dx = diff(path_x);
dy = diff(path_y);%计算差分

%用中点欧拉法要比向前欧拉法和向后欧拉法要更精确，但是也可能计算出的结果比精确值多一个pi
%在这里对dx,dy做中点欧拉法，使用四象限反正切计算角度

dx_pre = [dx(1);dx];
dx_after = [dx;dx(end)];
dx_final = (dx_pre + dx_after) / 2;

dy_pre = [dy(1);dy];
dy_after = [dy;dy(end)];
dy_final = (dy_pre + dy_after) / 2;

ds_final = sqrt(dx_final.^2 + dy_final.^2);
path_heading = atan2(dy_final,dx_final);

%atan2(b，a)：4象限反正切，

%　　　　计算b/a对应的反正切值，求点(a，b)对应的角
% 　　　　　(a，b)位于第一象限时，atan2(b，a)取值  0 ~ pi/2
% 　　　　　(a，b)位于第二象限时，atan2(b，a)取值  pi/2 ~ pi
% 　　　　　(a，b)位于第三象限时，atan2(b，a)取值   -pi ~ -pi/2
% 　　　　　(a，b)位于第四象限时，atan2(b，a)取值   -pi/2 ~ 0
%

%中点欧拉法
dheading = diff(path_heading);%差分，size变成length(path_heading) - 1
dheading_pre = [dheading(1);dheading]; %插入一个首元素
dheading_after = [dheading;dheading(end)]; %插入一个尾元素
dheading_final = (dheading_pre + dheading_after) / 2;
%为了防止dheading出现一个2*pi的错误，假设真实的heading较小，用sin(dheading)近似dheading
path_kappa = sin(dheading_final)./ds_final;

== matlab function testEmplanner_cs_old/Audi_A8_Sedan_1/decision&planning module/Subsystem/MATLAB Function2 ==
  data: host_match_point_index input; xr output; path_x input; path_y input; paht_heading input; path_kappa input; yr output; thetar output; kappa output
function [xr,yr,thetar,kappa] = fcn(host_match_point_index,path_x,path_y,paht_heading,path_kappa)
index = host_match_point_index(1);
xr = path_x(index + 1);
yr = path_y(index + 1);
thetar = paht_heading(index + 1);
kappa = path_kappa(index + 1);
%#codegen

== matlab function testEmplanner_cs_old/Audi_A8_Sedan_1/perception module/MATLAB Function ==
  data: host_x input; obs_x_set_gcs output; host_y input; host_heading_xy input; obs_range input; obs_theta input; obs_velocity input; obs_velocity_heading input; obs_y_set_gcs output; obs_velocity_set_gcs output; obs_heading_set_gcs output
function [obs_x_set_gcs,obs_y_set_gcs,obs_velocity_set_gcs,obs_heading_set_gcs] = ... 
	fcn(host_x,host_y,host_heading_xy,obs_range,obs_theta,obs_velocity,obs_velocity_heading)
 
 % gcs 全局坐标系 global coordinate system
 % 该函数是感知模块，输出障碍物的位置，速度大小 速度方向与世界坐标系x轴之间的夹角
 % 输入：定位信息 host_x,host_y，host_heading_xy 世界坐标系
 % 		 障碍物在传感器坐标系下的极坐标range，theta
 % 		 障碍物的速度大小 velocity
 %		 障碍物的速度方向与x轴的夹角 heading
 % 输出：障碍物在世界坐标系下的x y v v与x轴的夹角heading
 % 注意：注意输出得heading是障碍物的速度heading，不是障碍物的几何heading
  
 %传感器最多输出32个障碍物信息，但是事先不知道有多少个障碍物，所以要做个缓冲
 
 %输出初始化
 obs_x_set_gcs = ones(32,1)*nan;
 obs_y_set_gcs = ones(32,1)*nan;
 obs_velocity_set_gcs = ones(32,1)*nan;
 obs_heading_set_gcs = ones(32,1)*nan;
 %传感器极坐标的角度以顺时针为正，世界坐标是逆时针为正
 theta_transfer = -obs_theta * pi /180 ; %转化成弧度输出
 %velocity的方向以北为0度，世界坐标以东为0度。
 heading_transfer = (-obs_velocity_heading + 90*ones(32,1)) * pi / 180;
 % 计算障碍物到传感器的x方向距离，y方向的距离
 x_transfer = obs_range.* cos(theta_transfer + host_heading_xy);
 y_transfer = obs_range.* sin(theta_transfer + host_heading_xy);
 
 
 %计算障碍物的世界坐标
for i = 1 : 32
	if obs_range(i) ~= 0 
		obs_x_set_gcs(i) = x_transfer(i) + host_x + 2.16 * cos(host_heading_xy);
		obs_y_set_gcs(i) = y_transfer(i) + host_y + 2.16 * sin(host_heading_xy);
		obs_heading_set_gcs(i) = heading_transfer(i);
		obs_velocity_set_gcs(i) = obs_velocity(i);
	end
end

== matlab function testEmplanner_cs_old/Audi_A8_Sedan_1/control module/control main/longitudinal control double PID/MATLAB Function3 ==
  data: kp input; pid_out output; ki input; kd input; err input; err_delay input
function pid_out = fcn(kp,ki,kd,err,err_delay)

persistent integral;
if isempty(integral)
    integral = err * ki *0.01;
    devia = kd*(err - err_delay)/0.01;
    pid_out = kp*err + integral + devia;
else
    integral = integral + err * ki *0.01;
    devia = kd*(err - err_delay)/0.01;
    pid_out = kp*err + integral + devia;
end

== matlab function testEmplanner_cs_old/Audi_A8_Sedan_1/decision&planning module/EM Planner/path planning task/MATLAB Function ==
  data: dp_path_s input; l_min output; dp_path_l input; static_obs_s_set input; static_obs_l_set input; static_obs_length input; static_obs_width input; l_max output
function[l_min,l_max] = fcn(dp_path_s,dp_path_l,static_obs_s_set,static_obs_l_set,static_obs_length,static_obs_width)
%该函数将输出每个离散点的dp_path_s中的点s所对应的l的边界l_min,l_max
%输入:动态规划的曲线dp_path_s,dp_path_l
% 	 障碍物中心点的坐标static_obs_s_set,static_obs_l_set
%	 障碍物的长宽 static_obs_length,static_obs_width
%输出 l_min,l_max的上下界


%注意一般真实的障碍物投影到frenet后，长宽会变得扭曲，在这里近似用直角坐标系的static_obs_length,static_obs_width的值代替frenet坐标下的值
%所以此 emplanner不能处理参考线曲率过大的场景，量化指标为（R >= 200)
% 大曲率场景的避障，参考线模块，还有障碍物投影模块，速度规划模块要做很多特殊处理

% 输出初始化,如果没有边界默认给+-6,真实场景下，给的应该是道路的上下边界
l_min = ones(60,1) * -8;
l_max = ones(60,1) * 8;

    % 对每个障碍物做遍历
    for i = 1 : length(static_obs_s_set)
	    if isnan(static_obs_s_set(i))
		    break;
	    end
	    % 计算障碍物尾部和头部的s
	    obs_s_min = static_obs_s_set(i) - static_obs_length/2;
	    obs_s_max = static_obs_s_set(i) + static_obs_length/2;
	    % 找到obs_s_min,obs_s_max 在dp_path_s中的位置
	    start_index = FindNearIndex(dp_path_s,obs_s_min);
	    end_index = FindNearIndex(dp_path_s,obs_s_max);
    
	    %判断动态规划的dp_path_l,在障碍物的上面还是下面（path在obs上面即决策为向左绕，否则向右绕）
    
	    if start_index == 1 && end_index == 1
		continue;
		    %障碍物已经完全跑到了车的后面，完全没有必要去处理
	    end
    
	    %取障碍物的中心点作为判断
	    centre_index = FindNearIndex(dp_path_s,static_obs_s_set(i));
	    path_l = dp_path_l(centre_index);
    
	    if path_l > static_obs_l_set(i)
		    %意味着决策是向左绕过障碍物
		    for j = start_index : end_index
			    % l_min(j) 是所有决策为向左绕过障碍物的l的边界的最大值
			    l_min(j) = max(l_min(j),static_obs_l_set(i) + static_obs_width/2); 
		    end
	    else
		    % 意味着决策是向右绕过障碍物
		    for j = start_index:end_index
			    % l_max(j) 是所有决策为向右绕过障碍物的l的边界的最小值
			    l_max(j) = min(l_max(j),static_obs_l_set(i) - static_obs_width/2);
		    end   
	    end
    
    end
end

function y = FindNearIndex(dp_path_s,obs_s)
	%该函数将找到dp_path_s上所有点中，与obs_s最近的点，并返回该点在dp_path_s中的编号
	%这里要注意dp_path_s是动态规划中的点，是动态规划的结果，必然是大于等于0小于等于59的。
	%而obs_s是障碍物在整个referenceline上的投影所得到的坐标，所以obs_s可能小于0,也可能大于59
	if dp_path_s(1) >= obs_s 
		%障碍物在车的后面
		y = 1;
		return;
	elseif dp_path_s(end) <= obs_s
		%障碍物在车的前面很远的地方
		y = 60;
		return;
	else
		index = 1;
		while dp_path_s(index) < obs_s
			index = index + 1;
		end
		%循环退出的条件是dp_path_s(index) >= obs_s 判断一下index和index-1到底哪个点 离obs更近了
		if dp_path_s(index) - obs_s > obs_s - dp_path_s(index - 1)
			y = index - 1;
		else
			y = index;
		end
	end
end
